simulink model "FileLoggerTester"  (R2012b)
settings: Solver=FixedStepDiscrete  StartTime=0.0  StopTime=inf  FixedStep=0.001  RelTol=1e-3
undefined symbols (not defined in the file): macaddr
libraries: xpcethernetlib x2, xpcnetworkbufferlib x1, simulink x1, Lib_FileLogger x1, xpclib x1
settings Model: xpc_rtwmakecfg_data=_xpcetherlib__xpcether8255xlib__xpcetherGbElib__xpcnblib_  SimulationMode=external  BufferReuse=off  Creator=gilja  LastModifiedBy=gilja
settings OptimizationCC: BlockReduction=off  OptimizeBlockIOStorage=off  BufferReuse=off  ExpressionFolding=off  LocalBlockOutputs=off
settings HardwareCC: ProdIntDivRoundTo=Zero  ProdEndianess=LittleEndian  ProdHWDeviceType=Generic->32-bit x86 compatible
settings RTWCC: SystemTargetFile=xpctarget.tlc  TemplateMakefile=xpc_default_tmf  Description=xPC Target  ProcessScript=xpctarget_make_rtw_hook  RTWCompilerOptimization=On
settings xpcTargetCC: TargetFcnLib=ansi_tfl_table_tmw.mat  CodeReplacementLibrary=XPC_BLAS  ParMdlRefBuildCompliant=on  ConcurrentExecutionCompliant=on  CombineSignalStateStructs=off  GRTInterface=on  xPCTaskExecutionProfile=off  xPCRL32EventNumber=5000  RL32IRQSourceModifier=7  xPCIRQSourceBoard=Parallel_Port  xPCIOIRQSlot=0x378  xPCLoadParamSetFile=off  xPCConcurrentTasks=off  xPCEnableSFAnimation=off

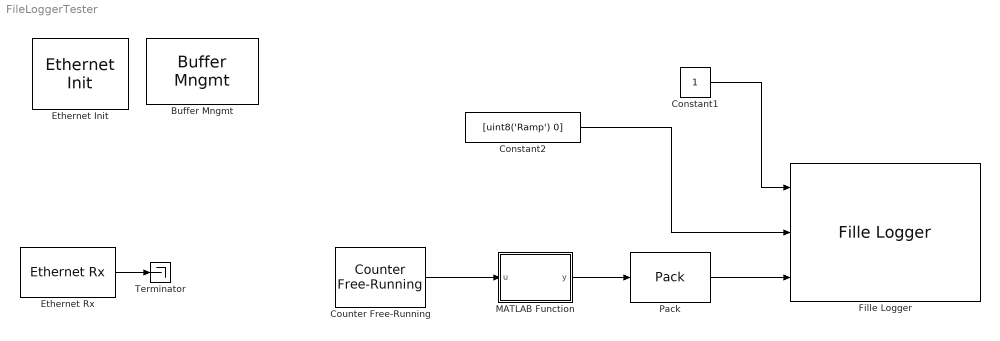
== system FileLoggerTester ==
  "Buffer Mngmt " : xpcnetworkbufferlib/Buffer Mngmt   Priority=-1  SampleTime=-1  PoolSizes=[100 10 10 200]  ShowTune=off
  Constant1 : Constant  OutDataTypeStr=uint8
  Constant2 : Constant  Value=[uint8('Ramp') 0]  OutDataTypeStr=uint8
  Counter Free-Running : simulink/Sources/Counter Free-Running  NumBits=32  tsamp=-1
  "Ethernet Init " : xpcethernetlib/Ethernet Init   Priority=-1  ID=1  Driver=Intel Gigabit  Bus=6  Slot=0  SampleTime=-1  AddressSource=EEPROM  MAC=macaddr('00:00:00:00:00:00')  TxSA=off  RxPromiscuous=off  Multicast={}  RxBad=off  RxShort=off  MaxMTU=1518  TxThreshold=224  TxBuffers=128  RxBuffers=64  ShowTune=off  NumRxBlks=1
  "Ethernet Rx " : xpcethernetlib/Ethernet Rx   ID=1  SampleTime=-1  Criteria=Receive all unmatched types [0 to 65535]  EtherType=[hex2dec('0000')]  BlkID=0
  Fille Logger : Lib_FileLogger/Fille Logger
  MATLAB Function : MATLAB Function  TreatAsAtomicUnit=on
  Pack : xpclib/UDP/Pack  datatypes={'uint32'}  byteAlign=1
  Terminator : Terminator
  wires:
  Constant1/1 -> Fille Logger/1
  Constant2/1 -> Fille Logger/2
  "Ethernet Rx "/1 -> Terminator/1
  Counter Free-Running/1 -> MATLAB Function/1(u)
  MATLAB Function/1(y) -> Pack/1
  Pack/1 -> Fille Logger/3

== matlab function FileLoggerTester/MATLAB Function ==
  data: u input; y output
function y = fcn(u)
%#codegen
y = uint32(zeros(1,200));

y(1:200) = u;
